simulink library "libBusSerialize"  (R2019a)
settings: Solver=ode45  StartTime=0.0  StopTime=10.0  RelTol=1e-3  EnableMultiTasking=on
undefined symbols (not defined in the file): BusSerialize, macaddr, mxpcnetworkconfig, RigInfo, SimulinkParameter_TestParamPulse, SimulinkParameter_TestParamToggle, SimulinkParameter_TunableConditions, SimulinkParameter_TunableNextTrialId, SimulinkParameter_TunableTaskControl, udpslgate
libraries: simulink x6, xpcethernetlib x3, xpcnetworkbufferlib x2, $bdroot x1
(part 1 of 2)
settings Model: xpc_rtwmakecfg_data=_xpcnblib__xpcetherlib__xpcether8255xlib__xpcetherGbElib__xpciplib_  Creator=Alexey Yu. Illarionov  LastModifiedBy=aillar
settings DataIOCC: LimitDataPoints=on  SaveFormat=Array
settings OptimizationCC: LifeSpan=inf
settings DebuggingCC: SolverPrmCheckMsg=warning  AllowSymbolicDim=off  PregeneratedLibrarySubsystemCodeDiagnostic=none  SFUnexpectedBacktrackingDiag=warning  SFNoUnconditionalDefaultTransitionDiag=warning  SFExecutionAtInitializationDiag=none  ArithmeticOperatorsInVariantConditions=warning
settings HardwareCC: ProdBitPerPointer=32  ProdBitPerSizeT=32  ProdBitPerPtrDiffT=32  ProdLargestAtomicFloat=None  ProdIntDivRoundTo=Undefined  ProdEndianess=Unspecified  ProdWordSize=32  ProdHWDeviceType=32-bit Generic
settings ModelReferenceCC: PropagateSignalLabelsOutOfModel=off
settings SFSimCC: SimUseLocalCustomCode=off
settings RTWCC: RTWUseLocalCustomCode=off
settings CodeAppCC: StateflowObjectComments=on
settings GRTTargetCC: TargetLangStandard=C89/C90 (ANSI)  GeneratePreprocessorConditionals=Disable all
settings ConfigComp: CovMetricSettings=dw  CovHtmlReporting=on  CovSaveCumulativeToWorkspaceVar=on  CovSaveSingleToWorkspaceVar=on  CovExternalEMLEnable=off  CovSFcnEnable=off

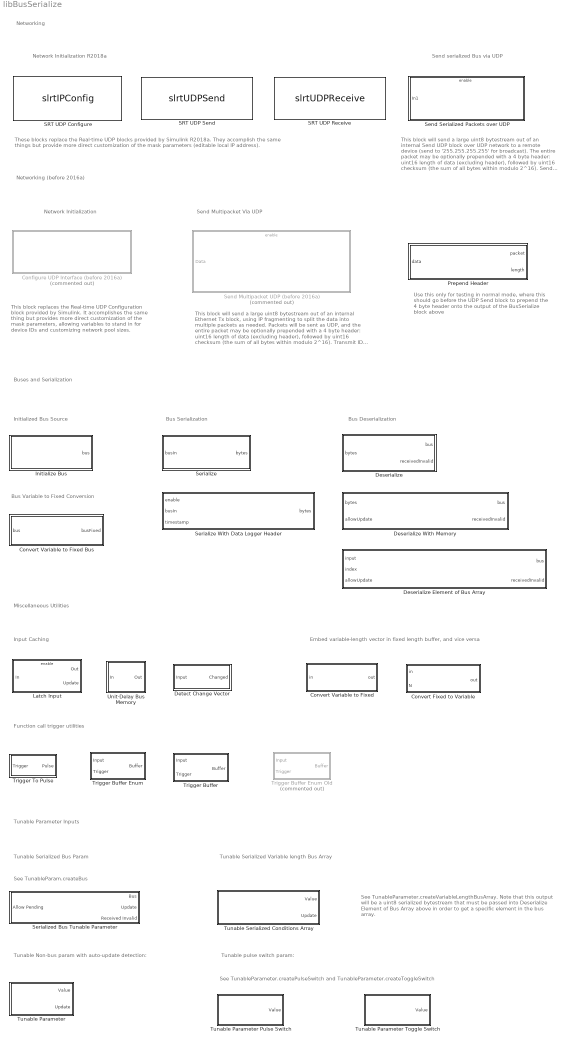
== system libBusSerialize ==
  note: See TunableParameter.createPulseSwitch and TunableParameter.createToggleSwitch
  note: See TunableParam.createBus
  note: See TunableParameter.createVariableLengthBusArray.
      | Note that this output will be a uint8 serialized bytestream that must
      | be passed into Deserialize Element of Bus Array above in order to get a
      | specific element in the bus array.
  note: Use this only for testing in normal mode,
      | where this should go before the UDP Send block
      | to prepend the 4 byte header onto the output of
      | the BusSerialize block above
  note: This block will send a large uint8 bytestream out of an internal Ethernet Tx block, using IP fragmenting to split the data into multiple packets as needed. Packets will be sent as UDP, and the entire packet may be optionally prepended with a 4 byte header: uint16 length of data (excluding header), followed by uint16 checksum (the sum of all bytes within modulo 2^16). Transmit ID must be unique for that ethernet card and is used by the receiving end to reassemble packets.
  note: Send Multipacket Via UDP
  note: Bus Serialization
  note: Bus Deserialization
  note: Bus Variable to Fixed Conversion
  note: Input Caching
  note: Function call trigger utilities
  note: Embed variable-length vector in fixed length buffer, and vice versa
  note: Initialized Bus Source
  note: Tunable Non-bus param with auto-update detection:
  note: Tunable pulse switch param:
  note: Tunable Serialized Bus Param
  note: Tunable Serialized Variable length Bus Array
  note: Network Initialization
  note: Networking (before 2016a)
  note: Buses and Serialization
  note: Miscellaneous Utilities
  note: Tunable Parameter Inputs
  note: This block replaces the Real-time UDP Configuration block provided by Simulink. It accomplishes the same thing but provides more direct customization of the mask parameters, allowing variables to stand in for device IDs and customizing network pool sizes.
  note: Networking
  note: These blocks replace the Real-time UDP blocks provided by Simulink R2018a. They accomplish the same things but provide more direct customization of the mask parameters (editable local IP address).
  note: Network Initialization R2018a
  note: This block will send a large uint8 bytestream out of an internal Send UDP block over UDP network to a remote device (send to '255.255.255.255' for broadcast).
      | The entire packet may be optionally prepended with a 4 byte header: uint16 length of data (excluding header), followed by uint16 checksum (the sum of all bytes within modulo 2^16).
      | Send width determines the width of the data input vector. If this value is less than the number of bytes in the packet, the excess bytes are discarded.
      | Note: Only one block with fixed combination Local IP address/Local port is allowed. Use -1 for Local port to have many blocks in the model.
  note: Send serialized Bus via UDP
  Configure UDP Interface (before 2016a) : Subsystem  Commented=on  InitFcn=mxpcnetworkconfig(1);  mask(xpcnwconfig){PoolSizes=[100 10 10 200], ID=RigInfo.network.someVLAN.ethernetId, udpID=0, IpAddress=RigInfo.network.someVLAN.sourceIP, SubnetMask=255.255.255.0, Gateway=0.0.0.0, EthDrv=Intel Gigabit, PciBus=RigInfo.network.someVLAN.pciBus, PciSlot=RigInfo.network.someVLAN.pciSlot}
      mask prompts: PoolSizes "Buffer pool sizes (256, 512, 1024, 2048):"; ID "Device ID:"; udpID "Internal UDP ID:"; IpAddress "IP Address:"; SubnetMask "Subnet Mask:"; EthDrv "Ethernet Driver:"; PciBus "PCI Bus:"; PciSlot "PCI Slot:"
      mask help: Configure network interface for real-time UDP communication
      mask init:
      | IpAddress = ipaddr(IpAddress);
      | SubnetMask = ipaddr(SubnetMask);
      | Gateway = ipaddr(Gateway);
      | set_param([gcb '/Ethernet Init '], 'ID', num2str(ID)); % update internal ID, we don't use promotion so the field can be text rather than popup
      | udpID = ID - 1;
      | [MaskDisplay] = mxpcnetworkconfig(2, ID, EthDrv, PciBus, PciSlot);
      | % set_param(gcb, 'MaskDisplay', MaskDisplay);
      mask Help: eval('xpcdoc(''RT_NETWORK_CONFIGURATION'')');
      mask TypeOptions PoolSizes: Buffer Mngmt /PoolSizes
      mask TypeOptions EthDrv: Ethernet Init /Driver
      mask DialogControl DescGroupVar Prompt: Real-Time UDP Configuration
      mask Display:
      | try
      |     ipStr = BusSerialize.ipStringFromAddress(IpAddress);
      |     disp(sprintf('Real-time UDP\nConfiguration\nPCI Bus: %d Slot: %d\nDevice ID: %d\nIP Address: %s', PciBus, PciSlot, ID, ipStr));
      | catch
      |     disp('Real-time UDP\nConfiguration');
      | end
  Convert Fixed to Variable : MATLAB Function  TreatAsAtomicUnit=on  mask(Converts Variable-size to fixed-size array){bufferSize=1500}
      mask prompts: bufferSize "Buffer Size"
      mask help: Specify maximum input size.
  Convert Variable to Fixed : MATLAB Function  TreatAsAtomicUnit=on  mask(Converts Variable-size to fixed-size array){bufferSize=1000}
      mask prompts: bufferSize "Buffer Size"
      mask help: Specify maximum input size.
  Convert Variable to Fixed Bus : MATLAB Function  TreatAsAtomicUnit=on  mask(Drop Variable Length Signals From Bus){busType=Bus: TestBus, busFixedType=Bus: TestBusFixed}
      mask prompts: busType "Bus Type (Input):"; busFixedType "Bus Type (Output):"
      mask help:
      | This block takes as input a bus with some variable length signals, drops all variable length signals from the bus and outputs a bus with the specified type (second drop-down). This is accomplished by calling the appropriate model packaged code function for this bus.
      |
      | See BusSerialize.createBusBaseWorkspaceWithFixedSizeSignalsOnly and BusSerialize.writeDropVariableLengthSignalsFromBusModelPackagedCode.
      mask init:
      | BusSerialize.maskDropVariableLengthSignalsFromBusBlockUpdate(gcb)
  Deserialize : MATLAB Function  TreatAsAtomicUnit=on  mask(BusSerialize: deserialize block){busType=Bus: TestBus}
      mask prompts: busType "Bus Type"
      mask help: Select the bus type below to deserialize into.
      mask init:
      | BusSerialize.maskDeserializeBlockUpdate(gcb)
  Deserialize Element of Bus Array : MATLAB Function  TreatAsAtomicUnit=on  mask(BusSerialize: deserialize a single element of a serialized bus array){busType=Bus: TestBus, inputVariable=off}
      mask prompts: busType "Bus Type:"; inputVariable "Input Variable Length"
      mask help:
      | Given a bus array serialized with BusSerialize.serializeVariableLengthBusArray, this block deserializes a specific element of that bus array. This allows bus arrays to be deserialized even when the bus contains variable length elements (or the array is of variable length), which implies that Simulink cannot currently handle the bus array.
      |
      | Select the bus type below to deserialize into.
      mask init:
      | BusSerialize.maskDeserializeVariableLengthBusArrayBlockUpdate(gcb)
  Deserialize With Memory : MATLAB Function  TreatAsAtomicUnit=on  mask(Deserialize Bus With Internal Memory){busType=Bus: TestBus}
      mask prompts: busType "Bus Type:"
      mask help:
      | This block deserializes a uint8 bytestream into a specific bus type. When the input changes, the block will deserialize the new input, and the deserialization is successful, it will internally store the updated bus.
      |
      | If allowUpdate is high at that point, the new bus value will be output immediately and update will be driven high. If not, pendingUpdate will be driven high, and the updated bus will be held in an internal persistent variable. When allowUpdate goes high, this updated bus will be passed to the output, and update will be driven high.
      |
      | If an invalid serialized bus is received, receivedInvalid will be driven high, and the bus output will not change from its previously stored value. If the initial value sent to this block is invalid, a default initialized bus will be output with all zeros or empty bus elements.
      mask init:
      | BusSerialize.maskDeserializeMemoryBlockUpdate(gcb);
  Detect Change Vector : Subsystem
  Initialize Bus : MATLAB Function  TreatAsAtomicUnit=on  mask(Initialize Bus Block){busType=Bus: TestBus}
      mask prompts: busType "Bus Type:"
      mask help: This block simply wraps an initializeBus_BusName() function and is useful for debugging where bus inputs are required. It acts essentially like a ground source for bus types.
      mask init:
      | BusSerialize.maskInitializeBusBlockUpdate(gcb);
  Latch Input : Subsystem  TreatAsAtomicUnit=on
  Prepend Header : MATLAB Function  TreatAsAtomicUnit=on  mask{prependHeader=on}
      mask prompts: prependHeader "Prepend Header"
  SRT UDP Configure : S-Function  Priority=-1  InitFcn=|  FunctionName=slrtIPConfig  Parameters=ipAdd, snMask, gwAdd, gwDest, enableMulticast, multicastAdd, multicastMask, PciBus, PciSlot, PciFunction, tune, 0  SFunctionDeploymentMode=off  EnableBusSupport=off  mask(slrtudpconfigure){IpAddress=RigInfo.network.someVLAN.sourceIP, SubnetMask=255.255.255.0, Gateway=0.0.0.0, PciBus=RigInfo.network.someVLAN.pciBus, PciSlot=RigInfo.network.someVLAN.pciSlot, PciFunction=RigInfo.network.someVLAN.pciFunction, ID=1, tune=0, enableMulticast=off, MulticastIpAddress={}, MulticastMask={}}
      | % Validate model
      | udpvalidatemodel(gcb);
      mask prompts: IpAddress "Local IP address:"; SubnetMask "Subnet mask:"; PciBus "PCI Bus:"; PciSlot "PCI Slot:"; PciFunction "PCI Function:"; ID "deviceID:"; enableMulticast "Enable multicast"; MulticastIpAddress "Multicast IP address list:"; MulticastMask "Mask:"
      mask help: Initialize Ethernet network interface to use for UDP communication in real-time applications.
      mask init:
      | % Validate mask parameter values
      | IpAddress = BusSerialize.ipStringFromAddress(IpAddress);
      | SubnetMask = BusSerialize.ipStringFromAddress(SubnetMask);
      | Gateway = BusSerialize.ipStringFromAddress(Gateway);
      | 
      | [ipAdd, snMask, gwAdd, gwDest, multicastAdd, multicastMask] = ...
      |     udpslgate('privateIPConfigure', 'validateParams', IpAddress, PciBus,...
      |     PciSlot, PciFunction, SubnetMask, Gateway, enableMulticast,...
      |     MulticastIpAddress, MulticastMask, 0);
      mask Help: eval('xpcdoc(''UDP_Configure'')');
      mask Callback enableMulticast: udpslgate('privateEnableMulticast',gcb)
      mask DialogControl DescGroupVar Prompt: UDP Configure
      mask DialogControl GeneralTabContainer Prompt: General
      mask DialogControl MuticastTabContainer Prompt: Multicast
      mask Display:
      | maskDisplay = udpslgate('privateIPConfigure', 'dispStr', IpAddress,...
      |     PciBus, PciSlot, PciFunction, SubnetMask, Gateway,...
      |     enableMulticast, MulticastIpAddress, MulticastMask, 0);
      | 
      | disp(maskDisplay)
      | 
      | if tune
      |     port_label('output', 1, 'Curr Free')
      |     port_label('output', 2, 'High Free')
      |     port_label('output', 3, 'Low Free')
      | end
  SRT UDP Receive : S-Function  LoadFcn=%udpslgate('privateupdateIPlist', gcb, 'LoadFcn');  InitFcn=|  FunctionName=slrtUDPReceive  Parameters=ipAddress, localPort, outWidth, useHostTargetComm, fmAdd, maxUDPQueue, rcvMulticast, multicastAdd, sampleTime  SFunctionDeploymentMode=off  EnableBusSupport=off  mask(slrtudpreceive){TO=RigInfo.network.someVLAN.toIP, ipAddress=[], ipAddressVal=Use host-target connection, localPort=RigInfo.network.someVLAN.toPort, rcvWidth=24, rcvFmAny=on, fmAddress=0.0.0.0, rcvMulticast=off, multicastAddress=[], maxUDPQueue=8, sampleTime=-1}
      | % Validate model
      | udpvalidatemodel(gcb);
      mask prompts: TO "Local IP address:"; ipAddress "Local IP address:"; ipAddressVal "Local IP address:"; localPort "Local port (1-65535):"; rcvWidth "Receive width (1-65504):"; rcvFmAny "Receive from any source"; fmAddress "From IP address:"; rcvMulticast "Receive multicast"; multicastAddress "Multicast group address:"; maxUDPQueue "Max packets in queue:"; sampleTime "Sample time (-1 for inherited):"
      mask help:
      | Receive data over UDP network from a remote device.
      |
      | 'Local IP address' applies only when the block executes on a target computer.
      mask init:
      | ipAddress = BusSerialize.ipStringFromAddress(TO);
      | 
      | % Validate mask parameter values
      | [fmAdd, outWidth, useHostTargetComm, multicastAdd] = ...
      |     udpslgate('privateUDPReceive', 'validateParams', ipAddress,...
      |     localPort, rcvWidth, rcvFmAny, fmAddress,...
      |     rcvMulticast, multicastAddress);
      mask Help: eval('xpcdoc(''UDP_Receive'')');
      mask Callback rcvFmAny: udpslgate('privateupdatevRcvFmAny', gcb)
      mask Callback rcvMulticast: udpslgate('privateReceiveMulticast', gcb)
      mask DialogControl DescGroupVar Prompt: UDP Receive
      mask Display:
      | try
      |   if strcmp(rcvFmAny, 'off')
      |     disp(sprintf('Receive UDP packets\nFrom: %s\n To: %s:%d', ...
      |       BusSerialize.ipStringFromAddress(fmAdd), ...
      |       BusSerialize.ipStringFromAddress(TO), localPort));
      |   else
      |     disp(sprintf('Receive UDP packets\nFrom: Any IP address\n To: %s:%d', ...
      |       BusSerialize.ipStringFromAddress(TO), localPort));
      |   end
      | catch
      |   disp('Receive UDP packets')
      | end
      | 
      | %maskDisplay = udpslgate('privateUDPReceive', 'dispStr', ipAddress, localPort,...
      | %    rcvWidth, rcvFmAny, fmAddress, rcvMulticast, multicastAddress);
      | %disp(maskDisplay)
      | 
      | port_label('output', 1, 'Data')
      | port_label('output', 2, 'Length')
  SRT UDP Send : S-Function  LoadFcn=%udpslgate('privateupdateIPlist', gcb, 'SetIPAddress');  InitFcn=|  FunctionName=slrtUDPSend  Parameters=ipAddress, localPort, toAdd, toPort, useHostTargetComm, sampleTime  SFunctionDeploymentMode=off  EnableBusSupport=off  mask(slrtudpsend){FROM=RigInfo.network.someVLAN.sourceIP, ipAddress=Use host-target connection, ipAddressVal=Use host-target connection, localPort=-1, TO=RigInfo.network.someVLAN.broadcastIP, toAddress=255.255.255.255, toPort=RigInfo.network.someVLAN.destPort, sampleTime=-1}
      | % Validate model
      | udpvalidatemodel(gcb);
      mask prompts: FROM "Local IP address:"; ipAddress "Local IP address:"; ipAddressVal "Local IP address:"; localPort "Local port (1-65535 | -1):"; TO "To IP address:"; toAddress "To IP address:"; toPort "To port (1-65535):"; sampleTime "Sample time (-1 for inherited):"
      mask help:
      | Send data over UDP network to a remote device. Send to 255.255.255.255 for broadcast. The value -1 for 'Local port' means that the block transmits using any available port.
      |
      | 'Local IP address' applies only when the block executes on a target computer.
      mask init:
      | % Update ipAddress popup options
      | %udpslgate('privateupdateIPlist', gcb, 'UpdateIPList');
      | 
      | ipAddress = BusSerialize.ipStringFromAddress(FROM);
      | toAddress = BusSerialize.ipStringFromAddress(TO);
      | 
      | % Validate mask parameter values
      | [toAdd, useHostTargetComm] = ...
      |   udpslgate('privateUDPSend', 'validateParams', ipAddress, localPort, toAddress, toPort);
      | 
      | if ~strcmp(ipAddress, 'Use host-target connection')
      |   useHostTargetComm = 0;
      | end
      settings: PreSaveFcn=%udpslgate('privateupdateIPlist', gcb, 'UpdateIpAddressVal');
      mask Help: eval('xpcdoc(''UDP_Send'')');
      mask DialogControl DescGroupVar Prompt: UDP Send
      mask Display:
      | try
      |   disp(sprintf('Send UDP packets\nFrom: %s:%d\n To: %s:%d', ...
      |     BusSerialize.ipStringFromAddress(FROM), localPort, ...
      |     BusSerialize.ipStringFromAddress(TO), toPort));
      | catch
      |   disp('Send UDP packets')
      | end
      | 
      | %maskDisplay = udpslgate('privateUDPSend', 'dispStr', ipAddress, localPort, toAddress, toPort);
      | %disp(maskDisplay)
      | 
      | port_label('input', 1, 'Data')
      | port_label('input', 2, 'Length')
  Send Multipacket UDP (before 2016a) : Subsystem  Commented=on  mask(Send Multipacket UDP Block){transmitId=1, sourceIP=[192 168 1 1], sourcePort=20000, destIP=[192 168 1 255], destPort=25000, destMac='ff:ff:ff:ff:ff:ff', deviceID=1, prependHeader=on}
      mask prompts: transmitId "Transmit ID (must be unique):"; sourceIP "Source IP:"; sourcePort "Source Port:"; destIP "Destination IP:"; destPort "Destination Port:"; destMac "Destination MAC:"; deviceID "Ethernet Device ID:"; prependHeader "Prepend 4-byte Header (uint16 length, uint16 checksum)"
      mask help: Splits a UDP packet into multiple pieces to be reassembled at the receiver
      mask init:
      | set_param([gcb, '/Packet Iterator/Ethernet Tx '], 'ID', num2str(deviceID));
      mask Display:
      | disp(sprintf('UDP Send Multipacket\nDevice ID: %d (Transmit %d)\nFrom: %s : %d\nTo: %s : %d\nDest Mac: %s', ...
      |     deviceID, transmitId, ...
      |     BusSerialize.ipStringFromAddress(sourceIP), sourcePort, ...
      |     BusSerialize.ipStringFromAddress(destIP), destPort, destMac));
      | port_label('input', 1, 'uint8');
      | port_label('Enable','Enable')
  Send Serialized Packets over UDP : Subsystem  LoadFcn=%udpslgate('privateupdateIPlist', gcb, 'SetIPAddress');  InitFcn=|  mask(Send Serialized UDP Packet Block){FROM=RigInfo.network.someVLAN.sourceIP, localPort=-1, TO=RigInfo.network.someVLAN.broadcastIP, toPort=RigInfo.network.someVLAN.destPort, bufferSize=65504, sampleTime=-1, prependHeader=on}
      | % Validate model
      | %udpvalidatemodel(gcb);
      mask prompts: FROM "Local IP address:"; localPort "Local port (1-65535 | -1):"; TO "To IP address:"; toPort "To port (1-65535):"; bufferSize "Send width (1-65504):"; sampleTime "Sample time (-1 for inherited):"; prependHeader "Prepend 4-byte Header (uint16 length, uint16 checksum)"
      mask help:
      | Send serialized Bus data over UDP network to a remote device. Send to '255.255.255.255' for broadcast. The value -1 for 'Local port' means that the block transmits using any available port.
      |
      | This block will send a large uint8 bytestream out of an internal Send UDP block.The entire packet may be optionally prepended with a 4 byte header: uint16 length of data (excluding header), followed by uint16 checksum (the sum of all bytes within modulo 2^16).
      |
      | Send width determines the width of the data input vector. If this value is less than the number of bytes in the packet, the excess bytes are discarded.
      mask init:
      | %ipAddress = BusSerialize.ipStringFromAddress(FROM);
      | %toAddress = BusSerialize.ipStringFromAddress(TO);
      | 
      | % Validate mask parameter values
      | %{
      | [toAdd, useHostTargetComm] = ...
      |     udpslgate('privateUDPSend', 'validateParams', ...
      |     BusSerialize.ipStringFromAddress(FROM), localPort, ...
      |     BusSerialize.ipStringFromAddress(TO), toPort);
      | %}
      | 
      | if prependHeader
      |   bufferSize = bufferSize + 4;
      | end
      | if bufferSize > 65504
      |   bufferSize = 65504;
      | end
      settings: PostSaveFcn=%udpslgate('privateupdateIPlist', gcb, 'UpdateIpAddressVal');
      mask Help: eval('xpcdoc(''UDP_Send'')');
      mask TypeOptions FROM: Send UDP Packet/UDP Send/FROM
      mask TypeOptions localPort: Send UDP Packet/UDP Send/localPort
      mask TypeOptions TO: Send UDP Packet/UDP Send/TO
      mask TypeOptions toPort: Send UDP Packet/UDP Send/toPort
      mask TypeOptions bufferSize: Send UDP Packet/Convert Variable to Fixed/bufferSize
      mask TypeOptions sampleTime: Send UDP Packet/UDP Send/sampleTime
      mask TypeOptions prependHeader: Send UDP Packet/Prepend Header/prependHeader
      mask Display:
      | try
      |   disp(sprintf('Send UDP packets\nFrom: %s:%d\n To: %s:%d', ...
      |     BusSerialize.ipStringFromAddress(FROM), localPort, ...
      |     BusSerialize.ipStringFromAddress(TO), toPort));
      | catch
      |   disp('Send UDP packets')
      | end
      | 
      | %maskDisplay = udpslgate('privateUDPSend', 'dispStr', ipAddress, localPort, toAddress, toPort);
      | %disp(maskDisplay)
      | 
      | port_label('input', 1, 'uint8');
      | port_label('Enable', 'Enable')
  Serialize : MATLAB Function  TreatAsAtomicUnit=on  mask(BusSerialize: serialize block){busType=Bus: TestBus}
      mask prompts: busType "Bus Type"
      mask help: Select the bus type below to serialize.
      mask init:
      | BusSerialize.maskSerializeBlockUpdate(gcb)
  Serialize With Data Logger Header : MATLAB Function  TreatAsAtomicUnit=on  mask(BusSerialize: serialize block){busType=Bus: TestBus, groupType=Control, groupName='groupName'}
      mask prompts: busType "Bus Type"; groupType "Group Type"; groupName "Group Name"
      mask help: Select the bus type below to serialize.
      mask init:
      | BusSerialize.maskSerializeWithDataLoggerHeaderBlockUpdate(gcb)
  Serialized Bus Tunable Parameter : Subsystem  mask(BusSerialize Tunable Parameter Block){paramName='TunableTaskControl'}
      mask prompts: paramName "Parameter Name"
      mask help: This block provides the value of a tunable Simulink.Parameter into the model. Since tunable parameters with xPC target can only be doubles, the functions BusSerialize.createTunableParameter and BusSerialize.setTunableParameter automatically handle typecasting and update counter insertion, and this block handles update detection, typecasting, and reshaping back to the original form. Currently, variable size parameters are not supported.
      mask init:
      | BusSerialize.maskSerializedBusTunableParameterBlockUpdate(gcb);
      mask Display:
      | port_label('output', 1, paramName);
      | port_label('output', 2, 'Update');
      | port_label('output', 3, 'Received Invalid');
      | port_label('input', 1, 'Allow Pending');
  Trigger Buffer : Subsystem  mask(Trigger Buffer){bufferSize=100}
      mask prompts: bufferSize "Buffer Size (elements)"
      mask help: This block concatenates all inputs it receives via a function-call trigger, with the output reflecting the concatenated inputs recevied during each single tick.
  Trigger Buffer Enum : Subsystem  mask(Trigger Buffer Enum){bufferType=Enum: EnumType, maxBufferSize=10}
      mask prompts: bufferType "Enum Type"; maxBufferSize "Max Buffer Size"
      mask help: This block concatenates all inputs it receives via a function-call trigger, with the output reflecting the concatenated inputs recevied during each single tick.
  Trigger Buffer Enum Old : Subsystem  Commented=on  mask(Trigger Buffer){bufferSize=10, bufferType=Enum: TaskEvent}
      mask prompts: bufferSize "Buffer Size (elements)"; bufferType "Enum Type"
      mask help: This block concatenates all inputs it receives via a function-call trigger, with the output reflecting the concatenated inputs recevied during each single tick.
  Trigger To Pulse : Subsystem  mask(Trigger to Pulse){}
      mask help: This block converts a function-call trigger to a single-tick pulse signal which can be used as an Enable input.
  Tunable Parameter : Subsystem  mask(BusSerialize Tunable Parameter Block){paramName='TunableParam'}
      mask prompts: paramName "Parameter Name"
      mask help: This block provides the value of a tunable Simulink.Parameter into the model. Since tunable parameters with xPC target can only be doubles, the functions BusSerialize.createTunableParameter and BusSerialize.setTunableParameter automatically handle typecasting and update counter insertion, and this block handles update detection, typecasting, and reshaping back to the original form. Currently, variable size parameters are not supported.
      mask init:
      | BusSerialize.maskTunableParameterBlockUpdate(gcb);
      mask Display:
      | port_label('output', 1, paramName)
      | port_label('output', 2, 'Update');
  Tunable Parameter Pulse Switch : Subsystem  mask(BusSerialize Tunable Parameter Block){paramName='TestParamPulse'}
      mask prompts: paramName "Parameter Name"
      mask help: This block provides the value of a tunable Simulink.Parameter into the model. Since tunable parameters with xPC target can only be doubles, the functions BusSerialize.createTunableParameter and BusSerialize.setTunableParameter automatically handle typecasting and update counter insertion, and this block handles update detection, typecasting, and reshaping back to the original form. Currently, variable size parameters are not supported.
      mask init:
      | BusSerialize.maskTunableParameterPulseSwitchBlockUpdate(gcb);
      settings: OpenFcn=|
      | paramName = getBlockParamEval(gcb, 'paramName');
      | param = BusSerialize.getTunableParameterReferenceFromName(paramName);
      | param.activatePulseSwitch();
      | 
      | % turn the block green
      | setBlockParam(gcb, 'BackgroundColor', 'green');
      | 
      | % wait a bit
      | pause(0.05);
      | 
      | % and set it back to white
      | setBlockParam(gcb, 'BackgroundColor', 'lightBlue');
      mask Display: port_label('output', 1, paramName)
  Tunable Parameter Toggle Switch : Subsystem  InitFcn=|  mask(BusSerialize Tunable Parameter Block){paramName='TestParamToggle'}
      | if ~isBlockInLibrary(gcb)
      |     paramName = getBlockParamEval(gcb, 'paramName');
      |     param = BusSerialize.getTunableParameterReferenceFromName(paramName);
      |     value = param.value;
      | 
      |     if value
      |         % turn the block green
      |         setBlockParam(gcb, 'BackgroundColor', 'green');  
      |     else
      |         % keep it white
      |         setBlockParam(gcb, 'BackgroundColor', 'lightBlue');
      |     end
      | end
      mask prompts: paramName "Parameter Name"
      mask help:
      | This block provides the value of a tunable Simulink.Parameter into the model. Since tunable parameters with xPC target can only be doubles, the functions BusSerialize.createTunableParameter and BusSerialize.setTunableParameter automatically handle typecasting and update counter insertion, and this block handles update detection, typecasting, and reshaping back to the original form. Currently, variable size parameters are not supported.
      |
      | Use BusSerialize.TunableParameter.create(paramName) to create a parameter with this name.
      mask init:
      | BusSerialize.maskTunableParameterToggleSwitchBlockUpdate(gcb);
      settings: OpenFcn=|
      | if ~isBlockInLibrary(gcb)
      |     paramName = getBlockParamEval(gcb, 'paramName');
      |     param = BusSerialize.getTunableParameterReferenceFromName(paramName);
      |     value = param.toggleSwitch();
      | else
      |     value = uint8(0);
      | end
      | 
      | if value
      |     % turn the block green
      |     setBlockParam(gcb, 'BackgroundColor', 'green');
      | else
      |     % keep it white
      |     setBlockParam(gcb, 'BackgroundColor', 'lightBlue');
      | end
      mask Display: port_label('output', 1, paramName)
  Tunable Serialized Conditions Array : Subsystem  mask(BusSerialize Tunable Parameter Variable Length Bus Array Block){paramName='TunableConditions'}
      mask prompts: paramName "Parameter Name"
      mask help:
      | This block provides the value of a tunable Simulink.Parameter into the model. Since tunable parameters with xPC target can only be doubles, the functions BusSerialize.createTunableParameter and BusSerialize.setTunableParameter automatically handle typecasting and update counter insertion, and this block handles update detection, typecasting, and reshaping back to the original form. Currently, variable size parameters are not supported.
      |
      | This block specifically extracts a serialized variable length bus array, which can then be passed into the variable length bus array element extractor block.
      mask init:
      | BusSerialize.maskTunableParameterVariableLengthBusArrayBlockUpdate(gcb);
      mask Display:
      | port_label('output', 1, paramName)
      | port_label('output', 2, 'Update');
  Unit-Delay Bus Memory : Subsystem  mask(Bus Unit-Delay Memory Block){busType=Bus: RigOutputBus}
      mask prompts: busType "Bus Type:"
      mask help: This block acts exactly like a Memory block and can be used to break algebraic loops. However, unlike Memory blocks, it supports bus signals with variable length bus elements. Internally, this is done by serializing the bus, passing it through a Memory block, and then deserializing at the other end.
      mask init:
      | BusSerialize.maskBusMemoryBlockUpdate(gcb);
      mask Display:
      | text(.5, 0.2, 'Bus Memory', 'HorizontalAlignment', 'center');
      | x = [0.5 0.7 0.7 0.3 0.3 0.25 NaN 0.35 0.3];
      | y = [0.4 0.4 0.8 0.8 0.4 0.45 NaN 0.45 0.4];
      | plot(x, y);

== system libBusSerialize/Configure UDP Interface (before 2016a) ==
  "ARP Init " : S-Function  Priority=0  FunctionName=xpcdebugarpinit  Parameters=Stats, Interface, IpAddress, SubnetMask, Gateway, EthernetId, Flags, BlockId, Retry, Timeout, Expiration, StaticAddressListIp, StaticAddressListMac, DiscoveryList, MulticastList, SampleTime  SFunctionDeploymentMode=off  EnableBusSupport=off  mask(arpinit){Interface=udpID, IpAddress=IpAddress, SubnetMask=SubnetMask, Gateway=Gateway, EthernetId=ID, BlockId=0, SampleTime=-1, Flags=hex2dec('00000697'), Stats=off, Retry=5, Timeout=20, Expiration=20*60, StaticAddressListIp=[], StaticAddressListMac=[], DiscoveryList=[], MulticastList=[]}
      mask prompts: IpAddress "IP Address"; SubnetMask "Subnet Mask"; EthernetId "Ethernet ID"; BlockId "Block ID"; SampleTime "Sample Time"; Stats "Statistics Port"; StaticAddressListIp "[Static IP]"; StaticAddressListMac "[Static MAC]"; DiscoveryList "[Discovery IP]"; MulticastList "[Multicast IP]"
      mask help: ARP Init
      mask init:
      | xpclinklib('xpciplib');
      mask Help: web('arpdebug.htm',  '-helpbrowser');
      mask DialogControl ParameterTabVar0 Prompt: ARP
      mask DialogControl ParameterTabVar01 Prompt: Advanced
      mask DialogControl ParameterTabVar012 Prompt: Timeouts
      mask DialogControl ParameterTabVar0123 Prompt: ARP Table
      mask DialogControl ParameterTabVar01234 Prompt: Multicast
      mask Display: disp('ARP Init');
  "Buffer Mngmt " : xpcnetworkbufferlib/Buffer Mngmt   Priority=-1  SampleTime=-1  PoolSizes=PoolSizes  ShowTune=off
      settings: SourceProductName=Simulink Real-Time  SourceProductBaseCode=XP
  "Ethernet Init " : xpcethernetlib/Ethernet Init   Priority=-1  ID=5  Driver=Intel Gigabit  Bus=PciBus  Slot=PciSlot  Function=0  SampleTime=-1  AddressSource=EEPROM  MAC=macaddr('00:00:00:00:00:00')  TxSA=off  RxPromiscuous=off  Multicast={}  RxBad=off  RxShort=off  MaxMTU=1518  TxThreshold=224  TxBuffers=128  RxBuffers=64  ShowTune=off  NumRxBlks=1
      settings: SourceProductName=Simulink Real-Time  SourceProductBaseCode=XP
  "IP Init " : S-Function  Priority=1  FunctionName=xpcdebugipinit  Parameters=Stats, Group, ArpId, IpAddress, SubnetMask, DefaultGateway, DefaultInterface, Flags, ToS, StartingId, TTL, SampleTime  SFunctionDeploymentMode=off  EnableBusSupport=off  mask(ipinit){Group=udpID, ArpId=[udpID], IpAddress=[IpAddress], SubnetMask=[SubnetMask], DefaultGateway=Gateway, DefaultInterface=0, SampleTime=-1, Flags=hex2dec('00000005'), ToS=hex2dec('00'), StartingId=10000, TTL=64, Stats=off}
      mask prompts: ArpId "[ARP ID]"; IpAddress "[IP Address]"; SubnetMask "[Subnet Mask]"; DefaultGateway "Default Gateway"; DefaultInterface "Default Interface"; SampleTime "Sample Time"; StartingId "Starting Id"; Stats "Statistics Port"
      mask help: IP Init
      mask init:
      | xpclinklib('xpciplib');
      mask Help: web('ipdebug.htm',  '-helpbrowser');
      mask DialogControl ParameterTabVar0 Prompt: IP
      mask DialogControl ParameterTabVar01 Prompt: Advanced
      mask Display: disp('IP Init');
  "UDP Init " : S-Function  Priority=2  FunctionName=xpcdebugudpinit  Parameters=Stats, Group, StartingPort, Flags, SampleTime  SFunctionDeploymentMode=off  EnableBusSupport=off  mask(udpinit){Group=udpID, StartingPort=10000, Flags=hex2dec('00000001'), SampleTime=-1, Stats=off}
      mask prompts: StartingPort "Starting Port"; SampleTime "Sample Time"; Stats "Statistics Port"
      mask help: UDP Init
      mask init:
      | xpclinklib('xpciplib');
      mask Help: web('udpdebug.htm',  '-helpbrowser');
      mask DialogControl ParameterTabVar0 Prompt: IP
      mask DialogControl ParameterTabVar01 Prompt: Advanced
      mask Display: disp('UDP Init');

== system libBusSerialize/Detect Change Vector ==
  Input : Inport
  Compare To Zero : simulink/Logic and Bit Operations/Compare To Zero  relop=~=  OutDataTypeStr=boolean
  Detect Change : simulink/Logic and Bit Operations/Detect Change  vinit=0  OutDataTypeStr=boolean
  Sum of Elements : Sum  Inputs=+
  Changed : Outport  OutDataTypeStr=uint8
  wires:
  Sum of Elements/1 -> Compare To Zero/1
  Detect Change/1 -> Sum of Elements/1
  Compare To Zero/1 -> Changed/1  "noteBusUpdate"
  Input/1 -> Detect Change/1

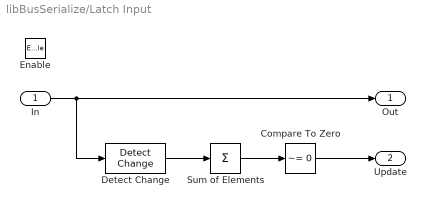
== system libBusSerialize/Latch Input ==
  In : Inport
  Enable : EnablePort
  Compare To Zero : simulink/Logic and Bit Operations/Compare To Zero  relop=~=  OutDataTypeStr=boolean  ZeroCross=off
  Detect Change : simulink/Logic and Bit Operations/Detect Change  vinit=0  OutDataTypeStr=boolean
  Sum of Elements : Sum  Inputs=+
  Out : Outport
  Update : Outport  Port=2  OutputWhenDisabled=reset  InitialOutput=0
  wires:
  In/1 -> Out/1, Detect Change/1
  Detect Change/1 -> Sum of Elements/1
  Sum of Elements/1 -> Compare To Zero/1
  Compare To Zero/1 -> Update/1

== system libBusSerialize/Send Multipacket UDP (before 2016a) ==
  Data : Inport  OutDataTypeStr=uint8
  Enable : EnablePort  PropagateVarSize=During execution
  Compare To Zero : simulink/Logic and Bit Operations/Compare To Zero  relop=>  OutDataTypeStr=boolean
  Packet Iterator : Subsystem
  Width : Width
  wires:
  Data/1 -> Packet Iterator/1(Data), Width/1
  Width/1 -> Compare To Zero/1
  Compare To Zero/1 -> Packet Iterator/Enable

== system libBusSerialize/Send Serialized Packets over UDP ==
  In1 : Inport
  Enable : EnablePort  PropagateVarSize=During execution
  Compare To Zero : simulink/Logic and Bit Operations/Compare To Zero  relop=>  OutDataTypeStr=boolean
  Send UDP Packet : Subsystem
  Width : Width  DataType=uint32
  wires:
  Compare To Zero/1 -> Send UDP Packet/Enable
  In1/1 -> Width/1, Send UDP Packet/1(In1)
  Width/1 -> Compare To Zero/1

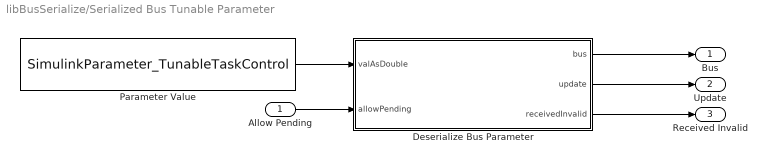
== system libBusSerialize/Serialized Bus Tunable Parameter ==
  Allow Pending : Inport
  Deserialize Bus Parameter : MATLAB Function  TreatAsAtomicUnit=on
  Parameter Value : Constant  Value=SimulinkParameter_TunableTaskControl  OutDataTypeStr=double
  Bus : Outport  PortDimensions=1
  Update : Outport  Port=2  OutDataTypeStr=uint8  PortDimensions=1
  Received Invalid : Outport  Port=3  OutDataTypeStr=uint8  PortDimensions=1
  wires:
  Deserialize Bus Parameter/2(update) -> Update/1
  Deserialize Bus Parameter/1(bus) -> Bus/1
  Deserialize Bus Parameter/3(receivedInvalid) -> Received Invalid/1
  Allow Pending/1 -> Deserialize Bus Parameter/2(allowPending)
  Parameter Value/1 -> Deserialize Bus Parameter/1(valAsDouble)

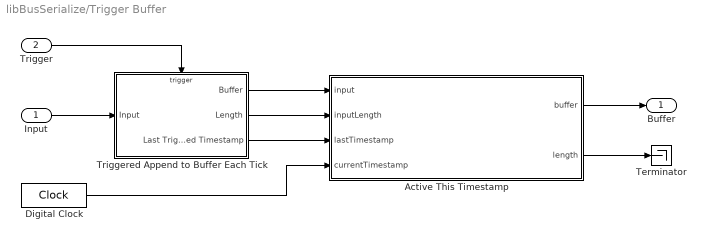
== system libBusSerialize/Trigger Buffer ==
  Input : Inport
  Trigger : Inport  Port=2
  Active This Timestamp : MATLAB Function  TreatAsAtomicUnit=on
  Digital Clock : DigitalClock  SampleTime=-1
  Terminator : Terminator
  Triggered Append to Buffer Each Tick : Subsystem
  Buffer : Outport
  wires:
  Active This Timestamp/2(length) -> Terminator/1
  Input/1 -> Triggered Append to Buffer Each Tick/1(Input)
  Triggered Append to Buffer Each Tick/3(Last Triggered Timestamp) -> Active This Timestamp/3(lastTimestamp)
  Triggered Append to Buffer Each Tick/2(Length) -> Active This Timestamp/2(inputLength)
  Triggered Append to Buffer Each Tick/1(Buffer) -> Active This Timestamp/1(input)
  Active This Timestamp/1(buffer) -> Buffer/1
  Digital Clock/1 -> Active This Timestamp/4(currentTimestamp)
  Trigger/1 -> Triggered Append to Buffer Each Tick/Trigger

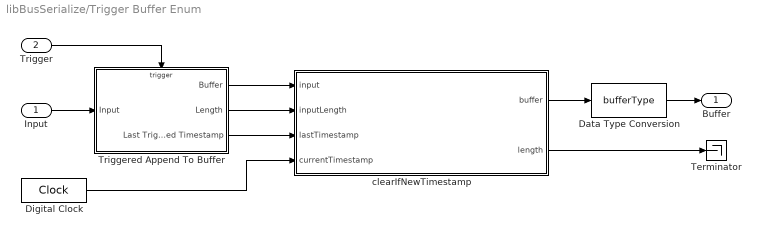
== system libBusSerialize/Trigger Buffer Enum ==
  Input : Inport  OutDataTypeStr=bufferType
  Trigger : Inport  Port=2
  Data Type Conversion : DataTypeConversion  OutDataTypeStr=bufferType
  Digital Clock : DigitalClock  SampleTime=-1
  Terminator : Terminator
  Triggered Append To Buffer : Subsystem
  clearIfNewTimestamp : MATLAB Function  TreatAsAtomicUnit=on
  Buffer : Outport  OutDataTypeStr=bufferType
  wires:
  Input/1 -> Triggered Append To Buffer/1(Input)
  clearIfNewTimestamp/1(buffer) -> Data Type Conversion/1
  Data Type Conversion/1 -> Buffer/1
  Trigger/1 -> Triggered Append To Buffer/Trigger
  Digital Clock/1 -> clearIfNewTimestamp/4(currentTimestamp)
  Triggered Append To Buffer/1(Buffer) -> clearIfNewTimestamp/1(input)
  Triggered Append To Buffer/2(Length) -> clearIfNewTimestamp/2(inputLength)
  Triggered Append To Buffer/3(Last Triggered Timestamp) -> clearIfNewTimestamp/3(lastTimestamp)
  clearIfNewTimestamp/2(length) -> Terminator/1

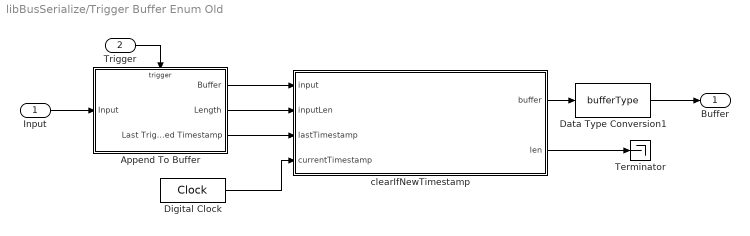
== system libBusSerialize/Trigger Buffer Enum Old ==
  Input : Inport  OutDataTypeStr=bufferType
  Trigger : Inport  Port=2
  Append To Buffer : Subsystem
  Data Type Conversion1 : DataTypeConversion  OutDataTypeStr=bufferType
  Digital Clock : DigitalClock  SampleTime=-1
  Terminator : Terminator
  clearIfNewTimestamp : MATLAB Function  TreatAsAtomicUnit=on
  Buffer : Outport  OutDataTypeStr=bufferType
  wires:
  Input/1 -> Append To Buffer/1(Input)
  clearIfNewTimestamp/1(buffer) -> Data Type Conversion1/1
  Data Type Conversion1/1 -> Buffer/1
  Trigger/1 -> Append To Buffer/Trigger
  Digital Clock/1 -> clearIfNewTimestamp/4(currentTimestamp)
  Append To Buffer/1(Buffer) -> clearIfNewTimestamp/1(input)
  Append To Buffer/2(Length) -> clearIfNewTimestamp/2(inputLen)
  Append To Buffer/3(Last Triggered Timestamp) -> clearIfNewTimestamp/3(lastTimestamp)
  clearIfNewTimestamp/2(len) -> Terminator/1

== system libBusSerialize/Trigger To Pulse ==
  Trigger : Inport
  Active This Timestamp : MATLAB Function  TreatAsAtomicUnit=on
  Capture timestamp : Subsystem
  Digital Clock : DigitalClock  SampleTime=-1
  Pulse : Outport
  wires:
  Active This Timestamp/1(active) -> Pulse/1
  Digital Clock/1 -> Active This Timestamp/2(currentTimestamp)
  Capture timestamp/1(Last Triggered Timestamp) -> Active This Timestamp/1(lastTimestamp)
  Trigger/1 -> Capture timestamp/Trigger

== system libBusSerialize/Tunable Parameter ==
  Deserialize Parameter : MATLAB Function  TreatAsAtomicUnit=on
  Parameter Value : Constant  Value=SimulinkParameter_TunableNextTrialId  OutDataTypeStr=double
  Value : Outport
  Update : Outport  Port=2
  wires:
  Deserialize Parameter/1(value) -> Value/1
  Deserialize Parameter/2(update) -> Update/1
  Parameter Value/1 -> Deserialize Parameter/1(valAsDouble)

== system libBusSerialize/Tunable Parameter Pulse Switch ==
  Deserialize Parameter : MATLAB Function  TreatAsAtomicUnit=on
  Parameter Value : Constant  Value=SimulinkParameter_TestParamPulse  OutDataTypeStr=double
  Terminator : Terminator
  Value : Outport  OutDataTypeStr=uint8  PortDimensions=1
  wires:
  Deserialize Parameter/1(value) -> Value/1
  Deserialize Parameter/2(update) -> Terminator/1
  Parameter Value/1 -> Deserialize Parameter/1(valAsDouble)

== system libBusSerialize/Tunable Parameter Toggle Switch ==
  Deserialize Parameter : MATLAB Function  TreatAsAtomicUnit=on
  Parameter Value : Constant  Value=SimulinkParameter_TestParamToggle  OutDataTypeStr=double
  Terminator : Terminator
  Value : Outport  OutDataTypeStr=uint8  PortDimensions=1
  wires:
  Deserialize Parameter/1(value) -> Value/1
  Deserialize Parameter/2(update) -> Terminator/1
  Parameter Value/1 -> Deserialize Parameter/1(valAsDouble)

== system libBusSerialize/Tunable Serialized Conditions Array ==
  Deserialize Parameter : MATLAB Function  TreatAsAtomicUnit=on
  Parameter Value : Constant  Value=SimulinkParameter_TunableConditions  OutDataTypeStr=double
  Value : Outport
  Update : Outport  Port=2
  wires:
  Parameter Value/1 -> Deserialize Parameter/1(valAsDouble)
  Deserialize Parameter/2(update) -> Update/1
  Deserialize Parameter/1(value) -> Value/1

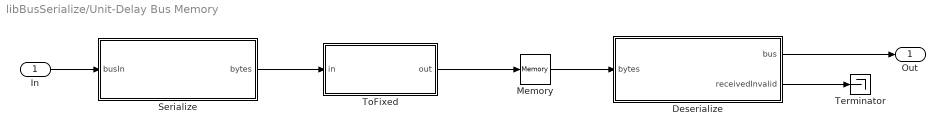
== system libBusSerialize/Unit-Delay Bus Memory ==
  In : Inport  OutDataTypeStr=Bus: RigOutputBus  PortDimensions=1
  Deserialize : MATLAB Function  TreatAsAtomicUnit=on  mask(BusSerialize: deserialize block){busType=Bus: RigOutputBus}
      mask prompts: busType "Bus Type"
      mask help: Select the bus type below to deserialize into.
      mask init:
      | BusSerialize.maskDeserializeBlockUpdate(gcb)
  Memory : Memory
  Serialize : MATLAB Function  TreatAsAtomicUnit=on  mask(BusSerialize: serialize block){busType=Bus: RigOutputBus}
      mask prompts: busType "Bus Type"
      mask help: Select the bus type below to serialize.
      mask init:
      | BusSerialize.maskSerializeBlockUpdate(gcb)
  Terminator : Terminator
  ToFixed : MATLAB Function  TreatAsAtomicUnit=on  mask(Converts Variable-size to fixed-size array){bufferSize=173164}
      mask prompts: bufferSize "Buffer Size"
      mask help: Specify maximum input size.
  Out : Outport  OutDataTypeStr=Bus: RigOutputBus
  wires:
  ToFixed/1(out) -> Memory/1
  Serialize/1(bytes) -> ToFixed/1(in)
  Memory/1 -> Deserialize/1(bytes)
  In/1 -> Serialize/1(busIn)
  Deserialize/2(receivedInvalid) -> Terminator/1
  Deserialize/1(bus) -> Out/1

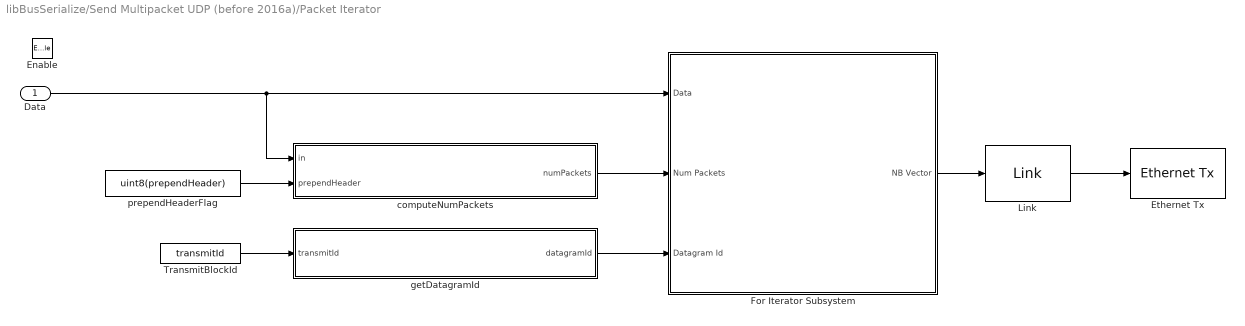
== system libBusSerialize/Send Multipacket UDP (before 2016a)/Packet Iterator ==
  Data : Inport
  Enable : EnablePort  PropagateVarSize=During execution
  "Ethernet Tx " : xpcethernetlib/Ethernet Tx   ID=1  SampleTime=-1
      settings: SourceProductName=Simulink Real-Time  SourceProductBaseCode=XP
  For Iterator Subsystem : Subsystem  TreatAsAtomicUnit=on
  "Link " : xpcnetworkbufferlib/Link 
      settings: SourceProductName=Simulink Real-Time  SourceProductBaseCode=XP
  TransmitBlockId : Constant  Value=transmitId  OutDataTypeStr=uint8
  computeNumPackets : MATLAB Function  TreatAsAtomicUnit=on
  getDatagramId : MATLAB Function  TreatAsAtomicUnit=on
  prependHeaderFlag : Constant  Value=uint8(prependHeader)  OutDataTypeStr=uint8
  wires:
  computeNumPackets/1(numPackets) -> For Iterator Subsystem/2(Num Packets)
  prependHeaderFlag/1 -> computeNumPackets/2(prependHeader)
  getDatagramId/1(datagramId) -> For Iterator Subsystem/3(Datagram Id)
  For Iterator Subsystem/1(NB Vector) -> "Link "/1
  TransmitBlockId/1 -> getDatagramId/1(transmitId)
  "Link "/1 -> "Ethernet Tx "/1
  Data/1 -> For Iterator Subsystem/1(Data), computeNumPackets/1(in)

== system libBusSerialize/Send Serialized Packets over UDP/Send UDP Packet ==
  In1 : Inport
  Enable : EnablePort  PropagateVarSize=During execution
  Convert Variable to Fixed : MATLAB Function  TreatAsAtomicUnit=on  mask(Converts Variable-size to fixed-size array){bufferSize=bufferSize}
      mask prompts: bufferSize "Buffer Size"
      mask help: Specify maximum input size.
  Data Type Conversion : DataTypeConversion  OutDataTypeStr=double
  Prepend Header : MATLAB Function  TreatAsAtomicUnit=on  mask{prependHeader=on}
      mask prompts: prependHeader "Prepend Header"
  UDP Send : $bdroot/SRT UDP Send  FROM=FROM  ipAddress=Use host-target connection  ipAddressVal=Use host-target connection  localPort=localPort  TO=TO  toAddress=255.255.255.255  toPort=toPort  sampleTime=sampleTime
  wires:
  In1/1 -> Prepend Header/1(data)
  Prepend Header/1(packet) -> Convert Variable to Fixed/1(in)
  Convert Variable to Fixed/1(out) -> UDP Send/1
  Prepend Header/2(length) -> Data Type Conversion/1
  Data Type Conversion/1 -> UDP Send/2

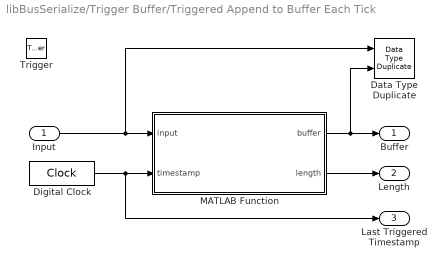
== system libBusSerialize/Trigger Buffer/Triggered Append to Buffer Each Tick ==
  Input : Inport
  Trigger : TriggerPort  TriggerType=function-call  VariantControl=Variant  StatesWhenEnabling=reset  PortDimensions=1
  Data Type Duplicate : DataTypeDuplicate
  Digital Clock : DigitalClock  SampleTime=-1
  MATLAB Function : MATLAB Function  TreatAsAtomicUnit=on
  Buffer : Outport
  Length : Outport  Port=2
  Last Triggered Timestamp : Outport  Port=3
  wires:
  Digital Clock/1 -> MATLAB Function/2(timestamp), Last Triggered Timestamp/1
  Input/1 -> MATLAB Function/1(input), Data Type Duplicate/1
  MATLAB Function/1(buffer) -> Buffer/1, Data Type Duplicate/2
  MATLAB Function/2(length) -> Length/1

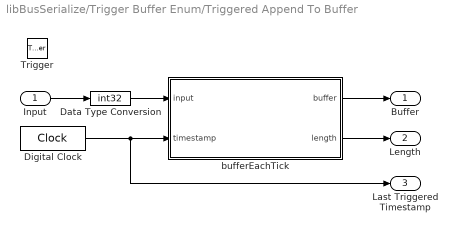
== system libBusSerialize/Trigger Buffer Enum/Triggered Append To Buffer ==
  Input : Inport  OutDataTypeStr=bufferType
  Trigger : TriggerPort  TriggerType=function-call  VariantControl=Variant  StatesWhenEnabling=reset  PortDimensions=1
  Data Type Conversion : DataTypeConversion  OutDataTypeStr=int32
  Digital Clock : DigitalClock  SampleTime=-1
  bufferEachTick : MATLAB Function  TreatAsAtomicUnit=on
  Buffer : Outport  OutDataTypeStr=int32
  Length : Outport  Port=2
  Last Triggered Timestamp : Outport  Port=3
  wires:
  bufferEachTick/2(length) -> Length/1
  bufferEachTick/1(buffer) -> Buffer/1
  Digital Clock/1 -> Last Triggered Timestamp/1, bufferEachTick/2(timestamp)
  Data Type Conversion/1 -> bufferEachTick/1(input)
  Input/1 -> Data Type Conversion/1

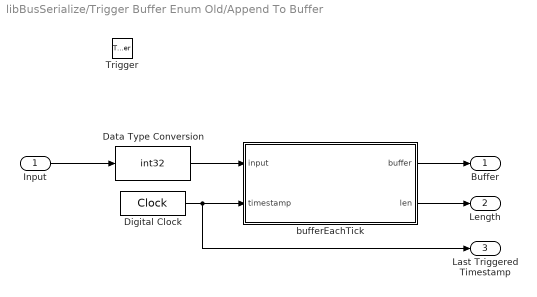
== system libBusSerialize/Trigger Buffer Enum Old/Append To Buffer ==
  Input : Inport  OutDataTypeStr=bufferType
  Trigger : TriggerPort  TriggerType=function-call  VariantControl=Variant  StatesWhenEnabling=reset  PortDimensions=1
  Data Type Conversion : DataTypeConversion  OutDataTypeStr=int32
  Digital Clock : DigitalClock  SampleTime=-1
  bufferEachTick : MATLAB Function  TreatAsAtomicUnit=on
  Buffer : Outport  OutDataTypeStr=int32
  Length : Outport  Port=2
  Last Triggered Timestamp : Outport  Port=3
  wires:
  bufferEachTick/2(len) -> Length/1
  bufferEachTick/1(buffer) -> Buffer/1
  Digital Clock/1 -> Last Triggered Timestamp/1, bufferEachTick/2(timestamp)
  Data Type Conversion/1 -> bufferEachTick/1(input)
  Input/1 -> Data Type Conversion/1

== system libBusSerialize/Trigger To Pulse/Capture timestamp ==
  Trigger : TriggerPort  TriggerType=function-call  VariantControl=Variant  StatesWhenEnabling=reset  PortDimensions=1
  Digital Clock : DigitalClock  SampleTime=-1
  Last Triggered Timestamp : Outport  OutputWhenDisabled=reset  InitialOutput=-1
  wires:
  Digital Clock/1 -> Last Triggered Timestamp/1

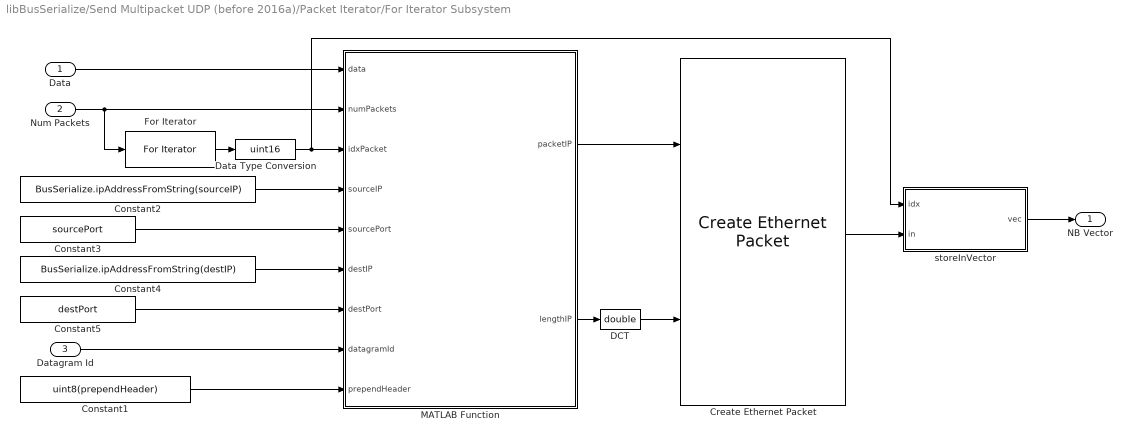
== system libBusSerialize/Send Multipacket UDP (before 2016a)/Packet Iterator/For Iterator Subsystem ==
  Data : Inport  OutDataTypeStr=uint8
  Num Packets : Inport  Port=2  OutDataTypeStr=uint16  PortDimensions=1
  Datagram Id : Inport  Port=3  OutDataTypeStr=uint8  PortDimensions=2
  Constant1 : Constant  Value=uint8(prependHeader)  OutDataTypeStr=uint8
  Constant2 : Constant  Value=BusSerialize.ipAddressFromString(sourceIP)  OutDataTypeStr=uint8
  Constant3 : Constant  Value=sourcePort  OutDataTypeStr=uint16
  Constant4 : Constant  Value=BusSerialize.ipAddressFromString(destIP)  OutDataTypeStr=uint8
  Constant5 : Constant  Value=destPort  OutDataTypeStr=uint16
  "Create Ethernet Packet " : xpcethernetlib/Create Ethernet Packet   DstMac=macaddr(destMac)  EtherType=hex2dec('0800')
      settings: SourceProductName=Simulink Real-Time  SourceProductBaseCode=XP
  DCT : DataTypeConversion  OutDataTypeStr=double
  Data Type Conversion : DataTypeConversion  OutDataTypeStr=uint16
  For Iterator : ForIterator  IterationSource=external  IterationVariableDataType=int16
  MATLAB Function : MATLAB Function  TreatAsAtomicUnit=on
  storeInVector : MATLAB Function  TreatAsAtomicUnit=on
  NB Vector : Outport
  wires:
  storeInVector/1(vec) -> NB Vector/1
  "Create Ethernet Packet "/1 -> storeInVector/2(in)
  Datagram Id/1 -> MATLAB Function/8(datagramId)
  Constant2/1 -> MATLAB Function/4(sourceIP)
  Constant3/1 -> MATLAB Function/5(sourcePort)
  Constant5/1 -> MATLAB Function/7(destPort)
  DCT/1 -> "Create Ethernet Packet "/2
  MATLAB Function/1(packetIP) -> "Create Ethernet Packet "/1
  MATLAB Function/2(lengthIP) -> DCT/1
  Constant1/1 -> MATLAB Function/9(prependHeader)
  Constant4/1 -> MATLAB Function/6(destIP)
  Data/1 -> MATLAB Function/1(data)
  Data Type Conversion/1 -> storeInVector/1(idx), MATLAB Function/3(idxPacket)
  Num Packets/1 -> For Iterator/1, MATLAB Function/2(numPackets)
  For Iterator/1 -> Data Type Conversion/1
